simulink model "numbertset"  (R2016b)
settings: Solver=VariableStepAuto  StartTime=0.0  StopTime=10.0  RelTol=1e-3
settings Model: Creator=E6320  LastModifiedBy=E6320

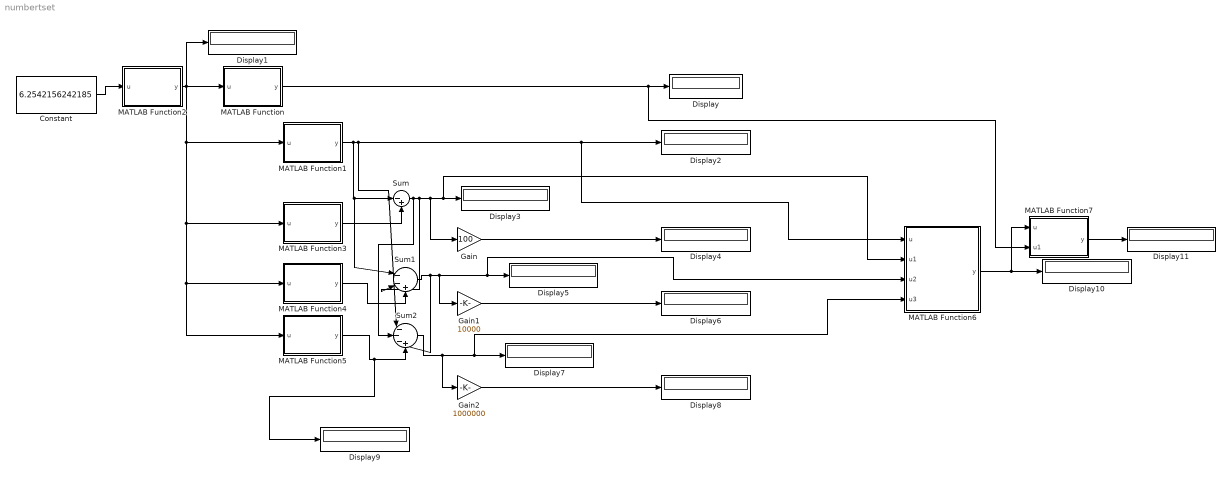
== system numbertset ==
  Constant : Constant  Value=6.2542156242185
  Display{,1..11} (12 alike) : Display
  Gain : Gain  Gain=100
  Gain1 : Gain  Gain=10000
  Gain2 : Gain  Gain=1000000
  MATLAB Function : MATLAB Function  TreatAsAtomicUnit=on
  MATLAB Function1 : MATLAB Function  TreatAsAtomicUnit=on
  MATLAB Function2 : MATLAB Function  TreatAsAtomicUnit=on
  MATLAB Function3 : MATLAB Function  TreatAsAtomicUnit=on
  MATLAB Function4 : MATLAB Function  TreatAsAtomicUnit=on
  MATLAB Function5 : MATLAB Function  TreatAsAtomicUnit=on
  MATLAB Function6 : MATLAB Function  TreatAsAtomicUnit=on
  MATLAB Function7 : MATLAB Function  TreatAsAtomicUnit=on
  Sum : Sum  Inputs=|-+
  Sum1 : Sum  Inputs=|--+
  Sum2 : Sum  Inputs=|---+
  wires:
  MATLAB Function/1(y) -> MATLAB Function7/2(u1), Display/1
  MATLAB Function2/1(y) -> MATLAB Function5/1(u), MATLAB Function4/1(u), MATLAB Function3/1(u), MATLAB Function1/1(u), Display1/1, MATLAB Function/1(u)
  Constant/1 -> MATLAB Function2/1(u)
  MATLAB Function1/1(y) -> Sum1/1, Sum/1, Sum2/1, MATLAB Function6/1(u), Display2/1
  Sum/1 -> Sum2/2, Sum1/2, Gain/1, MATLAB Function6/2(u1), Display3/1
  MATLAB Function3/1(y) -> Sum/2
  Gain/1 -> Display4/1
  MATLAB Function4/1(y) -> Sum1/3
  Gain1/1 -> Display6/1
  MATLAB Function5/1(y) -> Display9/1, Sum2/4
  Sum2/1 -> Gain2/1, MATLAB Function6/4(u3), Display7/1
  Gain2/1 -> Display8/1
  Sum1/1 -> Sum2/3, Gain1/1, MATLAB Function6/3(u2), Display5/1
  MATLAB Function6/1(y) -> MATLAB Function7/1(u), Display10/1
  MATLAB Function7/1(y) -> Display11/1

== matlab function numbertset/MATLAB Function1 ==
  data: u input; y output
function y = fcn(u)
y = abs(u)
y=floor(y);
end

== matlab function numbertset/MATLAB Function ==
  data: u input; y output
function y = fcn(u)
if(u<0)
y=99
elseif(u>0)
    y=88
else
    y=0
end

== matlab function numbertset/MATLAB Function2 ==
  data: u input; y output
function y = fcn(u)
y = floor(u*1000000)/1000000;
end

== matlab function numbertset/MATLAB Function3 ==
  data: u input; y output
function y = fcn(u)
y = abs(u)
y=floor(y*100)/100;
end

== matlab function numbertset/MATLAB Function4 ==
  data: u input; y output
function y = fcn(u)
y = abs(u)
y=floor(y*10000)/10000;
end

== matlab function numbertset/MATLAB Function5 ==
  data: u input; y output
function y = fcn(u)
y = abs(u)
y=floor(y*1000000)/1000000;
end

== matlab function numbertset/MATLAB Function6 ==
  data: u input; y output; u1 input; u2 input; u3 input
function y = fcn(u,u1,u2,u3)
y=u+u1+u2+u3
end

== matlab function numbertset/MATLAB Function7 ==
  data: u input; y output; u1 input
function y = fcn(u,u1)
if(u1==99)
y=-(u)
elseif(u1==88)
    y=u
else
    y=0
end
